simulink model "SPHERE_model3"  (R2020a)
settings: Solver=ode4  StartTime=0.0  StopTime=20  FixedStep=10e-4  RelTol=1e-3
values from neighbouring files (symbols this model uses):
  delay_r = 0.05    [Initial_script.m]    (also in Initial_script_test.m; Initial_script_test2.m)
  K = 25.937    [Initial_script.m]    (also in Initial_script_test.m; Initial_script_test2.m)
  L = -[ M2*l*(-2*l + R) - 2*J2, 0, -2*M2*l*g ]    [Initial_script.m]    (also in Initial_script_test.m; Initial_script_test2.m)
  L_trans = [A2-2*A3 0 -2*A4]    [Initial_script.m]    (also in Initial_script_test.m; Initial_script_test2.m)
  M = [ J1 + 2*J2 + M1*R^2 + M2*(2*l^2 - 3*R*l + R^2), -Tv, 2*l*g*M2 ]    [Initial_script.m]    (also in Initial_script_test.m; Initial_script_test2.m)
  M_trans = [A1 - 3*A2 + A3 -Tv 2*A4]    [Initial_script.m]    (also in Initial_script_test.m; Initial_script_test2.m)
  Smax = 502    [Initial_script.m]    (also in Initial_script_test.m; Initial_script_test2.m)
  Smin = -480    [Initial_script.m]    (also in Initial_script_test.m; Initial_script_test2.m)
  Top = 0.015    [Initial_script.m]    (also in Initial_script_test.m; Initial_script_test2.m)
  Tprob = 0.014    [Initial_script.m]    (also in Initial_script_test.m; Initial_script_test2.m)
libraries: simulink x1
settings Model: Creator=Adrian  LastModifiedBy=Adrian

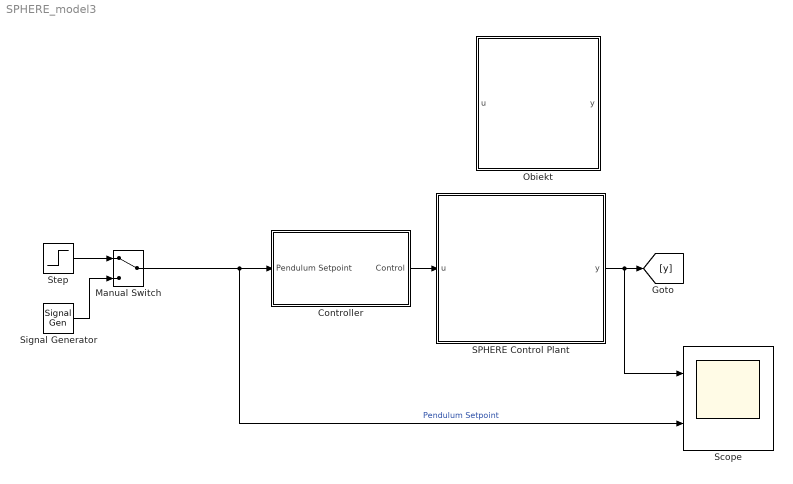
== system SPHERE_model3 ==
  Controller : Subsystem
  Manual Switch : ManualSwitch
  Obiekt : Subsystem
  SPHERE Control Plant : Subsystem
      mask Display: image('C:\Users\Adrian\Documents\Praca Magisterska\Robot kulisty by Adrian\Praca Magisterska\LaTex\Pictures\Old\sphere_full.PNG'); % Use "Edit Image" on toolstrip to change.
  Scope : Scope  NumInputPorts=2
  Signal Generator : SignalGenerator  WaveForm=square  Amplitude=45  Frequency=0.05
  Step : Step  Time=0.7  Before=60  After=0  SampleTime=0
  wires:
  SPHERE Control Plant/1(y) -> Scope/1, [y]
  Controller/1(Control) -> SPHERE Control Plant/1(u)
  Manual Switch/1 -> Controller/1(Pendulum Setpoint), Scope/2  "Pendulum Setpoint"
  Signal Generator/1 -> Manual Switch/2
  Step/1 -> Manual Switch/1

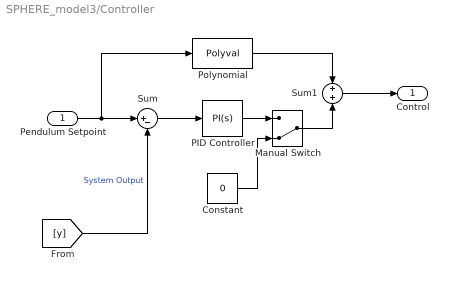
== system SPHERE_model3/Controller ==
  Pendulum Setpoint : Inport
  Constant : Constant  Value=0
  Manual Switch : ManualSwitch  CurrentSetting=0
  PID Controller : simulink/Continuous/PID Controller  Controller=PI  Form=Parallel  TimeDomain=Continuous-time  UseExternalTs=off  SampleTime=-1  IntegratorMethod=Forward Euler  FilterMethod=Forward Euler  ControllerParametersSource=internal  P=1  I=0  D=0  UseFilter=on  N=100  TunerSelectOption=Transfer Function Based (PID Tuner App)  InitialConditionSource=internal  InitialConditionForIntegrator=0  InitialConditionForFilter=0  DifferentiatorICPrevScaledInput=0  ExternalReset=none  TrackingMode=off  Kt=1  LimitOutput=off  UpperSaturationLimit=inf  LowerSaturationLimit=-inf  LinearizeAsGain=on  AntiWindupMode=none  Kb=1  POutMin=[]  POutMax=[]  IOutMin=[]  IOutMax=[]  DOutMin=[]  DOutMax=[]  NOutMin=[]  NOutMax=[]  SumOutMin=[]  SumOutMax=[]  SaturationOutMin=[]  SaturationOutMax=[]  PParamMin=[]  PParamMax=[]  IParamMin=[]  IParamMax=[]  DParamMin=[]  DParamMax=[]  NParamMin=[]  NParamMax=[]  KbParamMin=[]  KbParamMax=[]  KtParamMin=[]  KtParamMax=[]  KbOutMin=[]  KbOutMax=[]  KtOutMin=[]  KtOutMax=[]  IntegratorOutMin=[]  IntegratorOutMax=[]  FilterOutMin=[]  FilterOutMax=[]  SumI1OutMin=[]  SumI1OutMax=[]  SumI2OutMin=[]  SumI2OutMax=[]  SumI3OutMin=[]  SumI3OutMax=[]  SumI4OutMin=[]  SumI4OutMax=[]  SumDOutMin=[]  SumDOutMax=[]  DifferentiatorOutMin=[]  DifferentiatorOutMax=[]  FilterDiffOutCoefMin=[]  FilterDiffOutCoefMax=[]  ReciprocalOutMin=[]  ReciprocalOutMax=[]  SumDenOutMin=[]  SumDenOutMax=[]  SumNumOutMin=[]  SumNumOutMax=[]  DivideOutMin=[]  DivideOutMax=[]  UdiffTsProdOutMin=[]  UdiffTsProdOutMax=[]  NTsProdOutMin=[]  NTsProdOutMax=[]  UintegralTsProdOutMin=[]  UintegralTsProdOutMax=[]  UngainTsProdOutMin=[]  UngainTsProdOutMax=[]  IntegratorContinuousStateAttributes=''  IntegratorStateMustResolveToSignalObject=off  IntegratorRTWStateStorageClass=Auto  FilterContinuousStateAttributes=''  FilterStateMustResolveToSignalObject=off  FilterRTWStateStorageClass=Auto  ParallelPVariant=InternalParameters  IdealPVariant=Disabled  IVariant=InternalParameters  DVariant=Disabled  IntegratorVariant=Continuous  SatVariant=Disabled  AWVariant=Passthrough  PCopyVariant=Disabled  TRVariant=Disabled  FdbkBlocksVariant=Forward  IdealPFdbkVariant=Disabled  SatFdbkVariant=Disabled  DerivativeFilterVariant=Disabled  NVariant=Disabled  NCopyVariant=Disabled_SignalSpec  FilterICVariant=Disabled  IntegratorICVariant=InternalICs  ExternalResetVariant=Disabled  TRSumVariant=Passthrough  SumFdbkVariant=Disabled  SumVariant=Sum_PI  TsampFilterVariant=InternalTs  TsampNgainVariant=Passthrough  TsampIntegralVariant=Passthrough
  Polynomial : Polyval  Coefs=[0.000325 0.001274 1.044515 0]
  Sum : Sum  Inputs=|+-
  Sum1 : Sum  Inputs=+|+
  Control : Outport
  wires:
  Sum/1 -> PID Controller/1
  Polynomial/1 -> Sum1/1
  Pendulum Setpoint/1 -> Polynomial/1, Sum/1
  Manual Switch/1 -> Sum1/2
  [y] -> Sum/2  "System Output"
  Sum1/1 -> Control/1
  Constant/1 -> Manual Switch/2
  PID Controller/1 -> Manual Switch/1

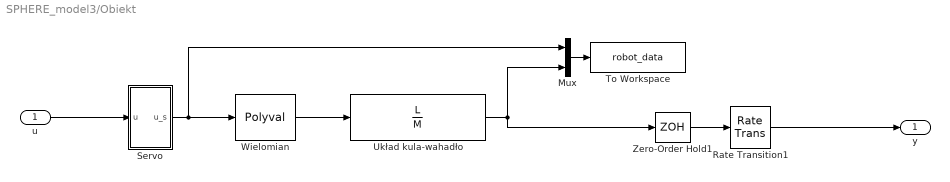
== system SPHERE_model3/Obiekt ==
  u : Inport
  Mux : Mux  Inputs=2
  Rate Transition1 : RateTransition
  Servo : Subsystem
  To Workspace : ToWorkspace  VariableName=robot_data  SaveFormat=Structure With Time  SampleTime=-1
  Układ kula-wahadło : TransferFcn  Numerator=L  Denominator=M
  Wielomian : Polyval  Coefs=[-0.000067 -0.000287 0.871698 0]
  Zero-Order Hold1 : ZeroOrderHold  SampleTime=Tprob
  y : Outport
  wires:
  u/1 -> Servo/1(u)
  Układ kula-wahadło/1 -> Mux/2, Zero-Order Hold1/1
  Servo/1(u_s) -> Wielomian/1, Mux/1
  Mux/1 -> To Workspace/1
  Zero-Order Hold1/1 -> Rate Transition1/1
  Rate Transition1/1 -> y/1
  Wielomian/1 -> Układ kula-wahadło/1

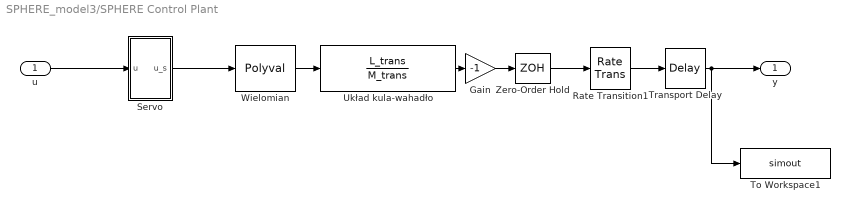
== system SPHERE_model3/SPHERE Control Plant ==
  u : Inport
  Gain : Gain  Gain=-1
  Rate Transition1 : RateTransition
  Servo : Subsystem
  To Workspace1 : ToWorkspace  VariableName=simout  SaveFormat=Timeseries  SampleTime=-1
  Transport Delay : TransportDelay  DelayTime=delay_r
  Układ kula-wahadło : TransferFcn  Numerator=L_trans  Denominator=M_trans
  Wielomian : Polyval  Coefs=[-0.000067 -0.000287 0.871698 0]
  Zero-Order Hold : ZeroOrderHold  SampleTime=Tprob
  y : Outport
  wires:
  u/1 -> Servo/1(u)
  Układ kula-wahadło/1 -> Gain/1
  Servo/1(u_s) -> Wielomian/1
  Wielomian/1 -> Układ kula-wahadło/1
  Gain/1 -> Zero-Order Hold/1
  Transport Delay/1 -> y/1, To Workspace1/1
  Zero-Order Hold/1 -> Rate Transition1/1
  Rate Transition1/1 -> Transport Delay/1

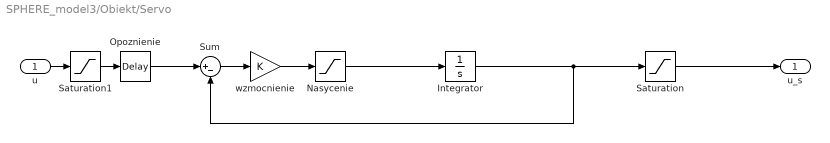
== system SPHERE_model3/Obiekt/Servo ==
  u : Inport
  Integrator : Integrator
  Nasycenie : Saturate  UpperLimit=Smax  LowerLimit=Smin
  Opoznienie : TransportDelay  DelayTime=Top
  Saturation : Saturate  UpperLimit=60  LowerLimit=-60
  Saturation1 : Saturate  UpperLimit=60  LowerLimit=-60
  Sum : Sum  Inputs=|+-
  wzmocnienie : Gain  Gain=K
  u_s : Outport
  wires:
  Sum/1 -> wzmocnienie/1
  Integrator/1 -> Saturation/1, Sum/2
  wzmocnienie/1 -> Nasycenie/1
  Opoznienie/1 -> Sum/1
  Nasycenie/1 -> Integrator/1
  u/1 -> Saturation1/1
  Saturation/1 -> u_s/1
  Saturation1/1 -> Opoznienie/1

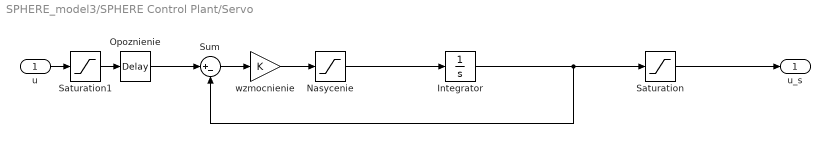
== system SPHERE_model3/SPHERE Control Plant/Servo ==
  u : Inport
  Integrator : Integrator
  Nasycenie : Saturate  UpperLimit=Smax  LowerLimit=Smin
  Opoznienie : TransportDelay  DelayTime=Top
  Saturation : Saturate  UpperLimit=60  LowerLimit=-60
  Saturation1 : Saturate  UpperLimit=60  LowerLimit=-60
  Sum : Sum  Inputs=|+-
  wzmocnienie : Gain  Gain=K
  u_s : Outport
  wires:
  Sum/1 -> wzmocnienie/1
  Integrator/1 -> Saturation/1, Sum/2
  wzmocnienie/1 -> Nasycenie/1
  Opoznienie/1 -> Sum/1
  Nasycenie/1 -> Integrator/1
  u/1 -> Saturation1/1
  Saturation/1 -> u_s/1
  Saturation1/1 -> Opoznienie/1
